simulink model "BP_MC1"  (Simulink 7.4)
settings: Solver=ode3  StartTime=0.0  StopTime=inf  FixedStep=0.05  RelTol=1e-3
libraries: simulink x2
settings Model: Creator=namdinh  LastModifiedBy=namdinh  BufferReuse=off
settings DataIOCC: SaveOutput=off  SignalLogging=off  SaveTime=off
settings OptimizationCC: BlockReduction=off  BooleanDataType=off  ConditionallyExecuteInputs=off  OptimizeBlockIOStorage=off  BufferReuse=off  ExpressionFolding=off  EnableMemcpy=off  LocalBlockOutputs=off  InitFltsAndDblsToZero=on
settings SFSimCC: SimBuildMode=sf_nonincremental_build
settings RTWCC: SystemTargetFile=nidll_vxworks.tlc  TemplateMakefile=nidll_vxworks.tmf  Description=NI Real-Time VxWorks Target for Release 2007b or later  ProcessScript=nidll_vxworks_make_rtw_hook
settings STFCustomTargetCC: GeneratePreprocessorConditionals=Disable all  MatFileLogging=on  SystemTargetFile=nidll_vxworks.tlc

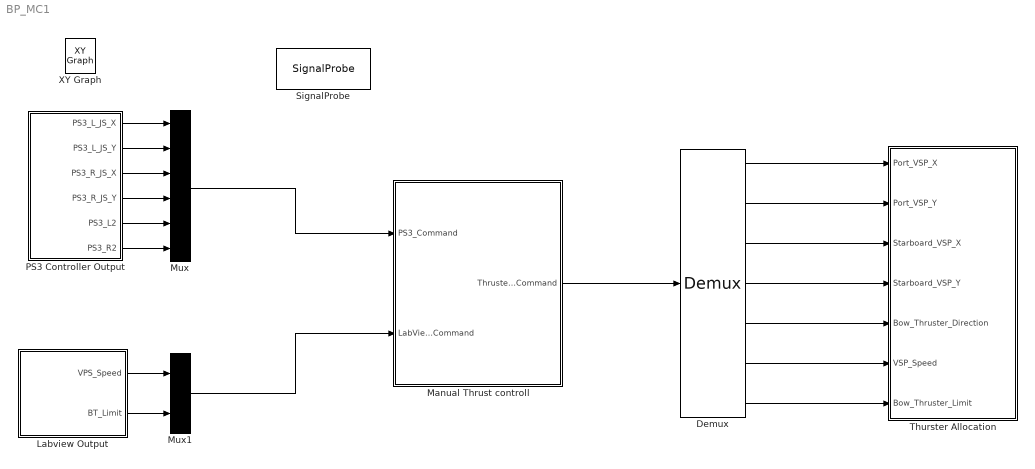
== system BP_MC1 ==
  Demux : Demux  Outputs=7
  Labview Output : Subsystem
  Manual Thrust controll : Subsystem
  Mux : Mux  Inputs=6
  Mux1 : Mux  Inputs=2
  PS3 Controller Output : Subsystem
  SignalProbe : S-Function  Description=Use this block with SIT.  FunctionName=SignalProbe  Parameters=1  EnableBusSupport=off
      settings: PreSaveFcn=NISIT_ModelVars;
      mask Description: The LabVIEW Simulation Interface Toolkit uses the SignalProbe block to probe the signals in the model. The SignalProbe block must be on the top level of the model hierarchy. You can have only one SignalProbe block per model file. Do not rename the SignalProbe block. Do not change the name of another model block to SignalProbe.
  Thurster Allocation : Subsystem
  XY Graph : simulink/Sinks/XY Graph  IOType=viewer  SystemSampleTime=-1  xmin=-1  xmax=1  ymin=-1  ymax=1  st=-1
  wires:
  PS3 Controller Output/1(PS3_L_JS_X) -> Mux/1
  PS3 Controller Output/2(PS3_L_JS_Y) -> Mux/2
  PS3 Controller Output/3(PS3_R_JS_X) -> Mux/3
  PS3 Controller Output/4(PS3_R_JS_Y) -> Mux/4
  PS3 Controller Output/5(PS3_L2) -> Mux/5
  PS3 Controller Output/6(PS3_R2) -> Mux/6
  Mux/1 -> Manual Thrust controll/1(PS3_Command)
  Labview Output/1(VPS_Speed) -> Mux1/1
  Labview Output/2(BT_Limit) -> Mux1/2
  Mux1/1 -> Manual Thrust controll/2(LabView_Command)
  Demux/1 -> Thurster Allocation/1(Port_VSP_X)
  Demux/2 -> Thurster Allocation/2(Port_VSP_Y)
  Demux/3 -> Thurster Allocation/3(Starboard_VSP_X)
  Demux/4 -> Thurster Allocation/4(Starboard_VSP_Y)
  Demux/5 -> Thurster Allocation/5(Bow_Thruster_Direction)
  Demux/6 -> Thurster Allocation/6(VSP_Speed)
  Demux/7 -> Thurster Allocation/7(Bow_Thruster_Limit)
  Manual Thrust controll/1(Thruster_Command) -> Demux/1

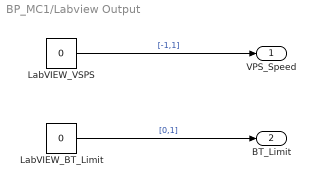
== system BP_MC1/Labview Output ==
  LabVIEW_BT_Limit : Constant  Value=0  OutDataType=fixdt(1, 16)  OutScaling=2^0
  LabVIEW_VSPS : Constant  Value=0  OutDataType=fixdt(1, 16)  OutScaling=2^0
  VPS_Speed : Outport  OutDataType=fixdt(1, 16)  OutScaling=2^0
  BT_Limit : Outport  Port=2  OutDataType=fixdt(1, 16)  OutScaling=2^0
  wires:
  LabVIEW_VSPS/1 -> VPS_Speed/1  "[-1,1]"
  LabVIEW_BT_Limit/1 -> BT_Limit/1  "[0,1]"

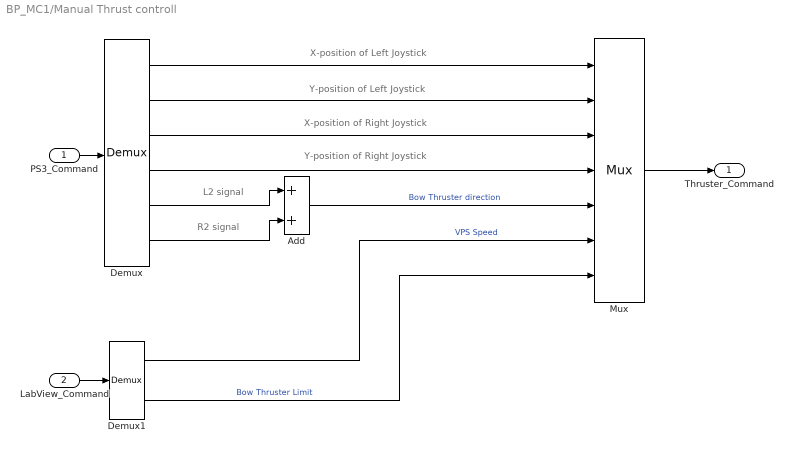
== system BP_MC1/Manual Thrust controll ==
  note: Y-position of Left Joystick
  note: X-position of Left Joystick
  note: X-position of Right Joystick
  note: Y-position of Right Joystick
  note: L2 signal
  note: R2 signal
  PS3_Command : Inport  OutDataType=fixdt(1, 16)  OutScaling=2^0
  LabView_Command : Inport  Port=2  OutDataType=fixdt(1, 16)  OutScaling=2^0
  Add : Sum  OutDataType=fixdt(1, 16)  OutScaling=2^-10
  Demux : Demux  Outputs=6
  Demux1 : Demux  Outputs=2
  Mux : Mux  Inputs=7
  Thruster_Command : Outport  OutDataType=fixdt(1, 16)  OutScaling=2^0
  wires:
  PS3_Command/1 -> Demux/1
  Demux/1 -> Mux/1
  Demux/2 -> Mux/2
  Demux/3 -> Mux/3
  Demux/4 -> Mux/4
  Demux/5 -> Add/1
  Demux/6 -> Add/2
  LabView_Command/1 -> Demux1/1
  Demux1/1 -> Mux/6  "VPS Speed"
  Demux1/2 -> Mux/7  "Bow Thruster Limit"
  Add/1 -> Mux/5  "Bow Thruster direction"
  Mux/1 -> Thruster_Command/1

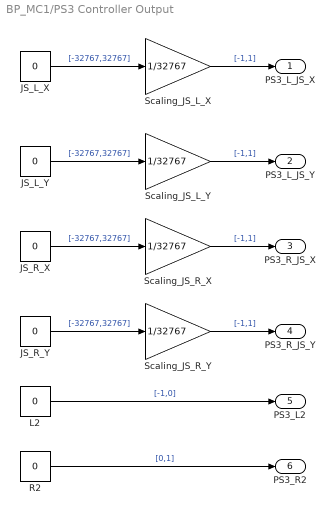
== system BP_MC1/PS3 Controller Output ==
  JS_L_X : Constant  Value=0  OutDataType=fixdt(1, 16)  OutScaling=2^0
  JS_L_Y : Constant  Value=0  OutDataType=fixdt(1, 16)  OutScaling=2^0
  JS_R_X : Constant  Value=0  OutDataType=fixdt(1, 16)  OutScaling=2^0
  JS_R_Y : Constant  Value=0  OutDataType=fixdt(1, 16)  OutScaling=2^0
  L2 : Constant  Value=0  OutDataType=fixdt(1, 16)  OutScaling=2^0
  R2 : Constant  Value=0  OutDataType=fixdt(1, 16)  OutScaling=2^0
  Scaling_JS_L_X : Gain  Gain=1/32767  ParameterDataType=fixdt(1, 16)  ParameterScaling=2^0  OutDataType=fixdt(1, 16)  OutScaling=2^0
  Scaling_JS_L_Y : Gain  Gain=1/32767  ParameterDataType=fixdt(1, 16)  ParameterScaling=2^0  OutDataType=fixdt(1, 16)  OutScaling=2^0
  Scaling_JS_R_X : Gain  Gain=1/32767  ParameterDataType=fixdt(1, 16)  ParameterScaling=2^0  OutDataType=fixdt(1, 16)  OutScaling=2^0
  Scaling_JS_R_Y : Gain  Gain=1/32767  ParameterDataType=fixdt(1, 16)  ParameterScaling=2^0  OutDataType=fixdt(1, 16)  OutScaling=2^0
  PS3_L_JS_X : Outport  OutDataType=fixdt(1, 16)  OutScaling=2^0
  PS3_L_JS_Y : Outport  Port=2  OutDataType=fixdt(1, 16)  OutScaling=2^0
  PS3_R_JS_X : Outport  Port=3  OutDataType=fixdt(1, 16)  OutScaling=2^0
  PS3_R_JS_Y : Outport  Port=4  OutDataType=fixdt(1, 16)  OutScaling=2^0
  PS3_L2 : Outport  Port=5  OutDataType=fixdt(1, 16)  OutScaling=2^0
  PS3_R2 : Outport  Port=6  OutDataType=fixdt(1, 16)  OutScaling=2^0
  wires:
  JS_L_X/1 -> Scaling_JS_L_X/1  "[-32767,32767]"
  Scaling_JS_L_X/1 -> PS3_L_JS_X/1  "[-1,1]"
  JS_L_Y/1 -> Scaling_JS_L_Y/1  "[-32767,32767]"
  Scaling_JS_L_Y/1 -> PS3_L_JS_Y/1  "[-1,1]"
  JS_R_X/1 -> Scaling_JS_R_X/1  "[-32767,32767]"
  Scaling_JS_R_X/1 -> PS3_R_JS_X/1  "[-1,1]"
  Scaling_JS_R_Y/1 -> PS3_R_JS_Y/1  "[-1,1]"
  JS_R_Y/1 -> Scaling_JS_R_Y/1  "[-32767,32767]"
  L2/1 -> PS3_L2/1  "[-1,0]"
  R2/1 -> PS3_R2/1  "[0,1]"

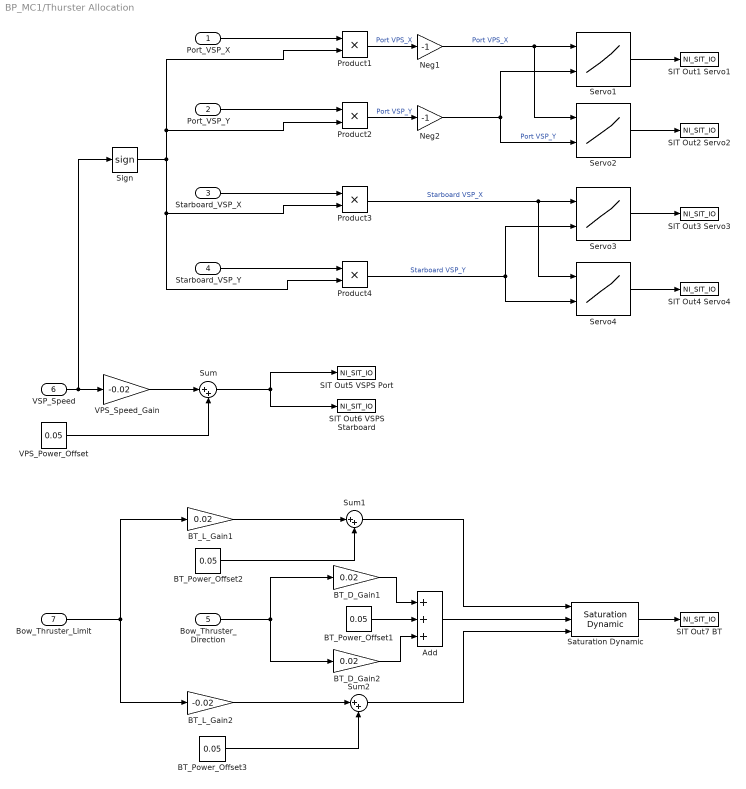
== system BP_MC1/Thurster Allocation ==
  Port_VSP_X : Inport  OutDataType=fixdt(1, 16)  OutScaling=2^0
  Port_VSP_Y : Inport  Port=2  OutDataType=fixdt(1, 16)  OutScaling=2^0
  Starboard_VSP_X : Inport  Port=3  OutDataType=fixdt(1, 16)  OutScaling=2^0
  Starboard_VSP_Y : Inport  Port=4  OutDataType=fixdt(1, 16)  OutScaling=2^0
  Bow_Thruster_Direction : Inport  Port=5  OutDataType=fixdt(1, 16)  OutScaling=2^0
  VSP_Speed : Inport  Port=6  OutDataType=fixdt(1, 16)  OutScaling=2^0
  Bow_Thruster_Limit : Inport  Port=7  OutDataType=fixdt(1, 16)  OutScaling=2^0
  Add : Sum  Inputs=+++  OutDataType=fixdt(1, 16)  OutScaling=2^-10
  BT_D_Gain1 : Gain  Gain=0.02  ParameterDataType=fixdt(1, 16)  ParameterScaling=2^0  OutDataType=fixdt(1, 16)  OutScaling=2^0
  BT_D_Gain2 : Gain  Gain=0.02  ParameterDataType=fixdt(1, 16)  ParameterScaling=2^0  OutDataType=fixdt(1, 16)  OutScaling=2^0
  BT_L_Gain1 : Gain  Gain=0.02  ParameterDataType=fixdt(1, 16)  ParameterScaling=2^0  OutDataType=fixdt(1, 16)  OutScaling=2^0
  BT_L_Gain2 : Gain  Gain=-0.02  ParameterDataType=fixdt(1, 16)  ParameterScaling=2^0  OutDataType=fixdt(1, 16)  OutScaling=2^0
  BT_Power_Offset1 : Constant  Value=0.05  OutDataType=fixdt(1, 16)  OutScaling=2^0
  BT_Power_Offset2 : Constant  Value=0.05  OutDataType=fixdt(1, 16)  OutScaling=2^0
  BT_Power_Offset3 : Constant  Value=0.05  OutDataType=fixdt(1, 16)  OutScaling=2^0
  Neg1 : Gain  Gain=-1  ParameterDataType=fixdt(1, 16)  ParameterScaling=2^0  OutDataType=fixdt(1, 16)  OutScaling=2^0
  Neg2 : Gain  Gain=-1  ParameterDataType=fixdt(1, 16)  ParameterScaling=2^0  OutDataType=fixdt(1, 16)  OutScaling=2^0
  Product{1..4} (4 alike) : Product  OutDataType=fixdt(1, 16)  OutScaling=2^0  RndMeth=Zero
  SIT Out1 Servo1 : S-Function  Priority=1  FunctionName=NI_SIT_IO  Parameters=width dtype portnum stime stype btype  EnableBusSupport=off  mask(SIT Outport){portnum=1, width=-1, stime=-1, dtype=auto, stype=auto, btype=0}
      mask prompts: portnum "Port number:"; width "Port dimensions (-1 for dynamically sized):"; stime "Sample time (-1 for inherited):"; dtype "Data type:"; stype "Signal type:"; btype "Block type:"
      mask help: Use this outport on any level of nested subsystems to allow the LabVIEW Simulation Interface Toolkit to map hardware to it.
      mask init:
      | NI_SIT_IO_init;
      settings: CopyFcn=NI_SIT_IO_callbacks(1);  DeleteFcn=NI_SIT_IO_callbacks(2);
      mask StyleString: edit,edit,edit,popup(auto|double|single|int8|uint8|int16|uint16|int32|uint32|boolean),popup(auto|real|complex),edit
      mask CallbackString: NI_SIT_IO_callbacks(3);|||NI_SIT_IO_callbacks(4);||
      mask TabNameString: Parameters,Parameters,Parameters,Parameters,Parameters,Parameters
      mask Display:
      | patch([-x x], [-y y], [.90980 .81960 .32156]);
      | plot([0 -x x 0], [rad -y y rad]);
      | fprintf('SIT%d', portnum);
  SIT Out2 Servo2 : S-Function  Priority=2  FunctionName=NI_SIT_IO  Parameters=width dtype portnum stime stype btype  EnableBusSupport=off  mask(SIT Outport){portnum=2, width=-1, stime=-1, dtype=auto, stype=auto, btype=0}
      mask prompts: portnum "Port number:"; width "Port dimensions (-1 for dynamically sized):"; stime "Sample time (-1 for inherited):"; dtype "Data type:"; stype "Signal type:"; btype "Block type:"
      mask help: Use this outport on any level of nested subsystems to allow the LabVIEW Simulation Interface Toolkit to map hardware to it.
      mask init:
      | NI_SIT_IO_init;
      settings: CopyFcn=NI_SIT_IO_callbacks(1);  DeleteFcn=NI_SIT_IO_callbacks(2);
      mask StyleString: edit,edit,edit,popup(auto|double|single|int8|uint8|int16|uint16|int32|uint32|boolean),popup(auto|real|complex),edit
      mask CallbackString: NI_SIT_IO_callbacks(3);|||NI_SIT_IO_callbacks(4);||
      mask TabNameString: Parameters,Parameters,Parameters,Parameters,Parameters,Parameters
      mask Display:
      | patch([-x x], [-y y], [.90980 .81960 .32156]);
      | plot([0 -x x 0], [rad -y y rad]);
      | fprintf('SIT%d', portnum);
  SIT Out3 Servo3 : S-Function  Priority=3  FunctionName=NI_SIT_IO  Parameters=width dtype portnum stime stype btype  EnableBusSupport=off  mask(SIT Outport){portnum=3, width=-1, stime=-1, dtype=auto, stype=auto, btype=0}
      mask prompts: portnum "Port number:"; width "Port dimensions (-1 for dynamically sized):"; stime "Sample time (-1 for inherited):"; dtype "Data type:"; stype "Signal type:"; btype "Block type:"
      mask help: Use this outport on any level of nested subsystems to allow the LabVIEW Simulation Interface Toolkit to map hardware to it.
      mask init:
      | NI_SIT_IO_init;
      settings: CopyFcn=NI_SIT_IO_callbacks(1);  DeleteFcn=NI_SIT_IO_callbacks(2);
      mask StyleString: edit,edit,edit,popup(auto|double|single|int8|uint8|int16|uint16|int32|uint32|boolean),popup(auto|real|complex),edit
      mask CallbackString: NI_SIT_IO_callbacks(3);|||NI_SIT_IO_callbacks(4);||
      mask TabNameString: Parameters,Parameters,Parameters,Parameters,Parameters,Parameters
      mask Display:
      | patch([-x x], [-y y], [.90980 .81960 .32156]);
      | plot([0 -x x 0], [rad -y y rad]);
      | fprintf('SIT%d', portnum);
  SIT Out4 Servo4 : S-Function  Priority=4  FunctionName=NI_SIT_IO  Parameters=width dtype portnum stime stype btype  EnableBusSupport=off  mask(SIT Outport){portnum=4, width=-1, stime=-1, dtype=auto, stype=auto, btype=0}
      mask prompts: portnum "Port number:"; width "Port dimensions (-1 for dynamically sized):"; stime "Sample time (-1 for inherited):"; dtype "Data type:"; stype "Signal type:"; btype "Block type:"
      mask help: Use this outport on any level of nested subsystems to allow the LabVIEW Simulation Interface Toolkit to map hardware to it.
      mask init:
      | NI_SIT_IO_init;
      settings: CopyFcn=NI_SIT_IO_callbacks(1);  DeleteFcn=NI_SIT_IO_callbacks(2);
      mask StyleString: edit,edit,edit,popup(auto|double|single|int8|uint8|int16|uint16|int32|uint32|boolean),popup(auto|real|complex),edit
      mask CallbackString: NI_SIT_IO_callbacks(3);|||NI_SIT_IO_callbacks(4);||
      mask TabNameString: Parameters,Parameters,Parameters,Parameters,Parameters,Parameters
      mask Display:
      | patch([-x x], [-y y], [.90980 .81960 .32156]);
      | plot([0 -x x 0], [rad -y y rad]);
      | fprintf('SIT%d', portnum);
  "SIT Out5 VSPS Port " : S-Function  Priority=41  FunctionName=NI_SIT_IO  Parameters=width dtype portnum stime stype btype  EnableBusSupport=off  mask(SIT Outport){portnum=41, width=-1, stime=-1, dtype=auto, stype=auto, btype=0}
      mask prompts: portnum "Port number:"; width "Port dimensions (-1 for dynamically sized):"; stime "Sample time (-1 for inherited):"; dtype "Data type:"; stype "Signal type:"; btype "Block type:"
      mask help: Use this outport on any level of nested subsystems to allow the LabVIEW Simulation Interface Toolkit to map hardware to it.
      mask init:
      | NI_SIT_IO_init;
      settings: CopyFcn=NI_SIT_IO_callbacks(1);  DeleteFcn=NI_SIT_IO_callbacks(2);
      mask StyleString: edit,edit,edit,popup(auto|double|single|int8|uint8|int16|uint16|int32|uint32|boolean),popup(auto|real|complex),edit
      mask CallbackString: NI_SIT_IO_callbacks(3);|||NI_SIT_IO_callbacks(4);||
      mask TabNameString: Parameters,Parameters,Parameters,Parameters,Parameters,Parameters
      mask Display:
      | patch([-x x], [-y y], [.90980 .81960 .32156]);
      | plot([0 -x x 0], [rad -y y rad]);
      | fprintf('SIT%d', portnum);
  SIT Out6 VSPS Starboard : S-Function  Priority=42  FunctionName=NI_SIT_IO  Parameters=width dtype portnum stime stype btype  EnableBusSupport=off  mask(SIT Outport){portnum=42, width=-1, stime=-1, dtype=auto, stype=auto, btype=0}
      mask prompts: portnum "Port number:"; width "Port dimensions (-1 for dynamically sized):"; stime "Sample time (-1 for inherited):"; dtype "Data type:"; stype "Signal type:"; btype "Block type:"
      mask help: Use this outport on any level of nested subsystems to allow the LabVIEW Simulation Interface Toolkit to map hardware to it.
      mask init:
      | NI_SIT_IO_init;
      settings: CopyFcn=NI_SIT_IO_callbacks(1);  DeleteFcn=NI_SIT_IO_callbacks(2);
      mask StyleString: edit,edit,edit,popup(auto|double|single|int8|uint8|int16|uint16|int32|uint32|boolean),popup(auto|real|complex),edit
      mask CallbackString: NI_SIT_IO_callbacks(3);|||NI_SIT_IO_callbacks(4);||
      mask TabNameString: Parameters,Parameters,Parameters,Parameters,Parameters,Parameters
      mask Display:
      | patch([-x x], [-y y], [.90980 .81960 .32156]);
      | plot([0 -x x 0], [rad -y y rad]);
      | fprintf('SIT%d', portnum);
  SIT Out7 BT : S-Function  Priority=43  FunctionName=NI_SIT_IO  Parameters=width dtype portnum stime stype btype  EnableBusSupport=off  mask(SIT Outport){portnum=43, width=-1, stime=-1, dtype=auto, stype=auto, btype=0}
      mask prompts: portnum "Port number:"; width "Port dimensions (-1 for dynamically sized):"; stime "Sample time (-1 for inherited):"; dtype "Data type:"; stype "Signal type:"; btype "Block type:"
      mask help: Use this outport on any level of nested subsystems to allow the LabVIEW Simulation Interface Toolkit to map hardware to it.
      mask init:
      | NI_SIT_IO_init;
      settings: CopyFcn=NI_SIT_IO_callbacks(1);  DeleteFcn=NI_SIT_IO_callbacks(2);
      mask StyleString: edit,edit,edit,popup(auto|double|single|int8|uint8|int16|uint16|int32|uint32|boolean),popup(auto|real|complex),edit
      mask CallbackString: NI_SIT_IO_callbacks(3);|||NI_SIT_IO_callbacks(4);||
      mask TabNameString: Parameters,Parameters,Parameters,Parameters,Parameters,Parameters
      mask Display:
      | patch([-x x], [-y y], [.90980 .81960 .32156]);
      | plot([0 -x x 0], [rad -y y rad]);
      | fprintf('SIT%d', portnum);
  Saturation Dynamic : simulink/Discontinuities/Saturation Dynamic  SystemSampleTime=-1  OutMin=[]  OutMax=[]  OutDataTypeStr=Inherit: Same as second input  OutDataType=fixdt(1, 16)  OutScaling=2^-10  DoSatur=off
  Servo1 : Lookup2D  RowIndex=[-1,0,1]  ColumnIndex=[-1,0,1]  Table=reshape([0.06,0.0495363,0.043301,0.06,0.052446,0.043301,0.06,0.0541518,0.043301],3,3)  OutDataType=fixdt(1, 16)  OutScaling=2^0
  Servo2 : Lookup2D  RowIndex=[-1,0,1]  ColumnIndex=[-1,0,1]  Table=reshape([0.03860880,0.0386088,0.03860880,0.0459941,0.0477243,0.0500953,0.057,0.057,0.057],3,3)  OutDataType=fixdt(1, 16)  OutScaling=2^0
  Servo3 : Lookup2D  RowIndex=[-1,0,1]  ColumnIndex=[-1,0,1]  Table=reshape([0.0640809,0.0640809,0.0640809,0.0539629,0.0541315,0.0556492,0.0442664,0.0442664,0.0442664],3,3)  OutDataType=fixdt(1, 16)  OutScaling=2^0
  Servo4 : Lookup2D  RowIndex=[-1,0,1]  ColumnIndex=[-1,0,1]  Table=reshape([0.0602867,0.0470489,0.0403879,0.0602867,0.049747,0.0403879,0.0602867,0.0526138,0.0403879],3,3)  OutDataType=fixdt(1, 16)  OutScaling=2^0
  Sign : Signum
  Sum : Sum  Inputs=|++  OutDataType=fixdt(1, 16)  OutScaling=2^0
  Sum1 : Sum  Inputs=|++  OutDataType=fixdt(1, 16)  OutScaling=2^0
  Sum2 : Sum  Inputs=|++  OutDataType=fixdt(1, 16)  OutScaling=2^0
  VPS_Power_Offset : Constant  Value=0.05  OutDataType=fixdt(1, 16)  OutScaling=2^0
  VPS_Speed_Gain : Gain  Gain=-0.02  ParameterDataType=fixdt(1, 16)  ParameterScaling=2^0  OutDataType=fixdt(1, 16)  OutScaling=2^0
  wires:
  Sign/1 -> Product1/2, Product2/2, Product3/2, Product4/2
  Product1/1 -> Neg1/1  "Port VPS_X"
  Product2/1 -> Neg2/1  "Port VSP_Y"
  Servo1/1 -> SIT Out1 Servo1/1
  Servo2/1 -> SIT Out2 Servo2/1
  Product3/1 -> Servo3/1, Servo4/1  "Starboard VSP_X"
  Product4/1 -> Servo3/2, Servo4/2  "Starboard VSP_Y"
  Servo3/1 -> SIT Out3 Servo3/1
  Servo4/1 -> SIT Out4 Servo4/1
  VSP_Speed/1 -> VPS_Speed_Gain/1, Sign/1
  VPS_Speed_Gain/1 -> Sum/1
  VPS_Power_Offset/1 -> Sum/2
  Sum/1 -> "SIT Out5 VSPS Port "/1, SIT Out6 VSPS Starboard/1
  Bow_Thruster_Direction/1 -> BT_D_Gain1/1, BT_D_Gain2/1
  BT_D_Gain1/1 -> Add/1
  BT_D_Gain2/1 -> Add/3
  BT_Power_Offset1/1 -> Add/2
  Add/1 -> Saturation Dynamic/2
  Bow_Thruster_Limit/1 -> BT_L_Gain1/1, BT_L_Gain2/1
  Sum1/1 -> Saturation Dynamic/1
  BT_L_Gain1/1 -> Sum1/1
  BT_L_Gain2/1 -> Sum2/1
  Sum2/1 -> Saturation Dynamic/3
  BT_Power_Offset2/1 -> Sum1/2
  BT_Power_Offset3/1 -> Sum2/2
  Saturation Dynamic/1 -> SIT Out7 BT/1
  Neg2/1 -> Servo1/2, Servo2/2  "Port VSP_Y"
  Neg1/1 -> Servo1/1, Servo2/1  "Port VPS_X"
  Starboard_VSP_Y/1 -> Product4/1
  Starboard_VSP_X/1 -> Product3/1
  Port_VSP_Y/1 -> Product2/1
  Port_VSP_X/1 -> Product1/1
